simulink model "cheetahSim"  (R2020b)
settings: Solver=ode23s  StartTime=0.0  StopTime=simTime  FixedStep=0.0005  MaxStep=0.001  RelTol=1e-8  AbsTol=1e-9
values from neighbouring files (symbols this model uses):
  A = [eye(3), zeros(3, 4)]    [cheetahAnim.m]    (also in cheetahEOM.m = jacobian(q(1:3), q); cheetahTrajOpt.m = [eye(3), zeros(3, 2)])
  Cd = 1.2    [cheetahTrajOpt.m]    (also in tailTrajOpt.m)
  p1_end__1 = [-l_t/2; 0; 0]    [cheetahAnim.m]    (also in cheetahEOM.m; tailAnim.m = [-L/2; 0; 0]; tailEOM.m = [-L/2; 0; 0])
  p_F = [pF1_1__1, pF1_2__1, pF2_1__2, pF2_2__2]    [cheetahAnim.m]
  p_s = [0; 0; 0.2 + h_b]    [cheetahAnim.m]    (also in cheetahEOM.m = [0; 0; 0])
  p_tb = [-l_b; 0; 0]    [cheetahAnim.m]    (also in cheetahEOM.m)
  tau_max = 30    [cheetahTrajOpt.m]    (also in tailTrajOpt.m)
  vert_b = [vert_b; vert_b - [l_b, 0, 0]]    [cheetahAnim.m]
libraries: simulink x7
settings Model: Creator=ricky  LastModifiedBy=ricky
settings SFSimCC: CustomCodeUndefinedFunction=UseInterfaceOnly

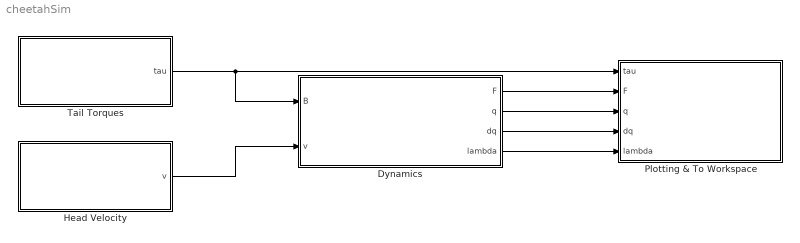
== system cheetahSim ==
  Dynamics : Subsystem
  Head Velocity : Subsystem
  Plotting & To Workspace : Subsystem
  Tail Torques : Subsystem
  wires:
  Dynamics/2(q) -> Plotting & To Workspace/3(q)
  Tail Torques/1(tau) -> Dynamics/1(B), Plotting & To Workspace/1(tau)
  Dynamics/1(F) -> Plotting & To Workspace/2(F)
  Dynamics/4(lambda) -> Plotting & To Workspace/5(lambda)
  Head Velocity/1(v) -> Dynamics/2(v)
  Dynamics/3(dq) -> Plotting & To Workspace/4(dq)

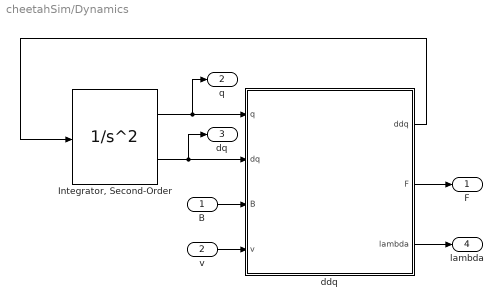
== system cheetahSim/Dynamics ==
  B : Inport
  v : Inport  Port=2
  "Integrator, Second-Order" : SecondOrderIntegrator  ICX=q0  ICDXDT=dq0
  ddq : MATLAB Function  TreatAsAtomicUnit=on
  F : Outport
  q : Outport  Port=2
  dq : Outport  Port=3
  lambda : Outport  Port=4
  wires:
  "Integrator, Second-Order"/2 -> dq/1, ddq/2(dq)
  "Integrator, Second-Order"/1 -> q/1, ddq/1(q)
  B/1 -> ddq/3(B)
  ddq/2(F) -> F/1
  ddq/3(lambda) -> lambda/1
  ddq/1(ddq) -> "Integrator, Second-Order"/1
  v/1 -> ddq/4(v)

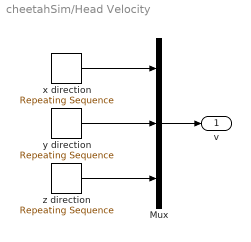
== system cheetahSim/Head Velocity ==
  Mux : Mux  Inputs=3
  x direction : simulink/Sources/Repeating Sequence  rep_seq_t=time  rep_seq_y=vx
  y direction : simulink/Sources/Repeating Sequence  rep_seq_t=time  rep_seq_y=vy
  z direction : simulink/Sources/Repeating Sequence  rep_seq_t=time  rep_seq_y=vz
  v : Outport
  wires:
  x direction/1 -> Mux/1
  y direction/1 -> Mux/2
  z direction/1 -> Mux/3
  Mux/1 -> v/1

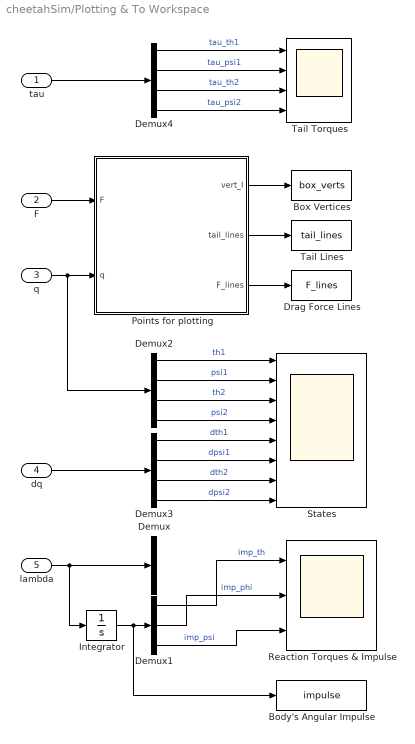
== system cheetahSim/Plotting & To Workspace ==
  tau : Inport
  F : Inport  Port=2
  q : Inport  Port=3
  dq : Inport  Port=4
  lambda : Inport  Port=5
  Body's Angular Impulse : ToWorkspace  VariableName=impulse  SampleTime=-1
      settings: Save2DSignal=2-D array (concatenate along first dimension)
  Box Vertices : ToWorkspace  VariableName=box_verts  SampleTime=-1
  Demux : Demux  Outputs=3
  Demux1 : Demux  Outputs=3
  Demux2 : Demux
  Demux3 : Demux
  Demux4 : Demux
  Drag Force Lines : ToWorkspace  VariableName=F_lines  SampleTime=-1
  Integrator : Integrator
  Points for plotting : MATLAB Function  TreatAsAtomicUnit=on
  Reaction Torques & Impulse : Scope  NumInputPorts=3
  States : Scope  NumInputPorts=8
  "Tail Lines " : ToWorkspace  VariableName=tail_lines  SampleTime=-1
  Tail Torques : Scope  NumInputPorts=4
  wires:
  F/1 -> Points for plotting/1(F)
  Points for plotting/1(vert_I) -> Box Vertices/1
  Points for plotting/2(tail_lines) -> "Tail Lines "/1
  Points for plotting/3(F_lines) -> Drag Force Lines/1
  Demux2/1 -> States/1  "th1"
  Demux3/3 -> States/7  "dth2"
  Demux2/4 -> States/4  "psi2"
  Demux3/4 -> States/8  "dpsi2"
  Demux3/1 -> States/5  "dth1"
  q/1 -> Demux2/1, Points for plotting/2(q)
  Demux3/2 -> States/6  "dpsi1"
  Demux2/3 -> States/3  "th2"
  dq/1 -> Demux3/1
  Demux2/2 -> States/2  "psi1"
  lambda/1 -> Integrator/1, Demux/1
  Demux1/1 -> Reaction Torques & Impulse/1  "imp_th"
  Demux1/3 -> Reaction Torques & Impulse/3  "imp_psi"
  Demux1/2 -> Reaction Torques & Impulse/2  "imp_phi"
  Integrator/1 -> Demux1/1, Body's Angular Impulse/1
  Demux4/2 -> Tail Torques/2  "tau_psi1"
  Demux4/1 -> Tail Torques/1  "tau_th1"
  Demux4/4 -> Tail Torques/4  "tau_psi2"
  Demux4/3 -> Tail Torques/3  "tau_th2"
  tau/1 -> Demux4/1

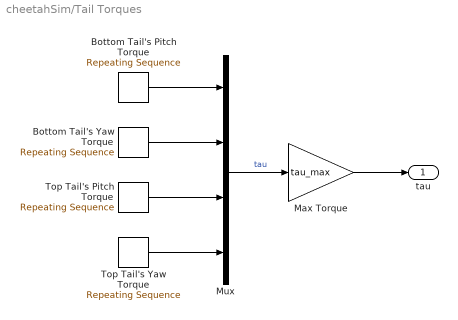
== system cheetahSim/Tail Torques ==
  Bottom Tail's Pitch Torque : simulink/Sources/Repeating Sequence  rep_seq_t=time_tau  rep_seq_y=tau1_th
  Bottom Tail's Yaw Torque : simulink/Sources/Repeating Sequence  rep_seq_t=time_tau  rep_seq_y=tau1_psi
  Max Torque : Gain  Gain=tau_max
  Mux : Mux
  Top Tail's Pitch Torque : simulink/Sources/Repeating Sequence  rep_seq_t=time_tau  rep_seq_y=tau2_th
  Top Tail's Yaw Torque : simulink/Sources/Repeating Sequence  rep_seq_t=time_tau  rep_seq_y=tau2_psi
  tau : Outport
  wires:
  Bottom Tail's Pitch Torque/1 -> Mux/1
  Bottom Tail's Yaw Torque/1 -> Mux/2
  Top Tail's Pitch Torque/1 -> Mux/3
  Top Tail's Yaw Torque/1 -> Mux/4
  Mux/1 -> Max Torque/1  "tau"
  Max Torque/1 -> tau/1

== matlab function cheetahSim/Plotting & To Workspace/Points for plotting ==
  data: F input; q input; p_F parameter; vert_I output; tail_lines output; p_s parameter; p_tb parameter; p1_end__1 parameter; vert_b parameter; F_lines output
function [vert_I, tail_lines, F_lines] = points4plot(F, q, p_F, p_s, p_tb, p1_end__1, vert_b)
    
    % rotation matrices
    R_I__b = RotZ(q(3)) * RotX(q(2)) * RotY(q(1));
    R_b__I = R_I__b';
    R_I__1 = RotZ(q(5)) * RotY(q(4)) * R_I__b;
    R_1__I = R_I__1'; % Rotation of bottom tail into body
    R_2__I = (RotZ(q(7)) * RotY(q(6)) * R_I__1)';

    % box vertex locations
    vert_I = zeros(8,3);
    for idx = 1:8
        vert_I(idx, :) = (p_s + R_b__I * vert_b(idx, :)')';
    end
    
    % tail point locations
    p_tb__I   = p_s + R_b__I*p_tb;
    p1_end__I = p_tb__I + R_1__I * p1_end__1;
    p2_end__I = p1_end__I + R_2__I * p1_end__1;

    tail1 = [p_tb__I, p1_end__I];
    tail2 = [p1_end__I, p2_end__I];
    tail_lines = reshape([tail1, tail2], [3, 2, 2]);
    
    % drag force locations
    pF1_1__I = p_tb__I + R_1__I * p_F(:, 1);
    pF1_2__I = p_tb__I + R_1__I * p_F(:, 2);
    pF2_1__I = p1_end__I + R_2__I * p_F(:, 3);
    pF2_2__I = p1_end__I + R_2__I * p_F(:, 4);
    
    F  = F/10;
    f1 = [pF1_1__I-F(:, 1), F(:, 1)];
    f2 = [pF1_2__I-F(:, 2), F(:, 2)];
    f3 = [pF2_1__I-F(:, 3), F(:, 3)];
    f4 = [pF2_2__I-F(:, 4), F(:, 4)];
    F_lines = reshape([f1, f2, f3, f4], [3, 2, 4]);
end
function rot = RotX(th)
    rot = [[1     0       0   ]
           [0  cos(th) sin(th)]
           [0 -sin(th) cos(th)]];
end
% function rot = RotY(th) % standard rotation about y
%     rot = [[ cos(th) 0 sin(th)]
%            [    0    1    0   ]
%            [-sin(th) 0 cos(th)]];
% end
function rot = RotY(th) % Liam's rotation about y
    rot = [[ cos(th) 0 -sin(th)]
           [    0    1    0   ]
           [sin(th) 0 cos(th)]];
end
function rot = RotZ(th)
    rot = [[ cos(th) sin(th) 0]
           [-sin(th) cos(th) 0]
           [    0       0    1]];
end

== matlab function cheetahSim/Dynamics/ddq ==
  data: ddq output; F output; lambda output; q input; dq input; B input; A parameter; Cd parameter; v input
function [ddq, F, lambda]  = ddq( q, dq, B, A, Cd, v)
    coder.extrinsic('cheetahMCGQ');
    coder.extrinsic('cheetahDragForces');
    
    F1_1 = zeros(3, 1);
    F1_2 = F1_1;
    F2_1 = F1_1;
    F2_2 = F1_1;
    [F1_1, F1_2, F2_1, F2_2] = cheetahDragForces(q, dq, Cd, v);
    F = [F1_1, F1_2, F2_1, F2_2];
    
    B = [zeros(3, 1); B];
    M = zeros(7, 7);
    C = zeros(7, 1);
    G = C;
    Q = C;
    [M, C, G, Q] = cheetahMCGQ(q, dq, F);
    lambda = -(A*(M\A'))\(A*(M\(B-C-G)));
    
    ddq = M\(B + Q + A'*lambda - G - C);
end
